simulink model "MPU6050_real_time_Kalman"  (R2023a)
settings: Solver=FixedStepAuto  StartTime=0.0  StopTime=30  RelTol=1e-3
libraries: arduinosensorlib x1
settings Model: ExtModeTrigDuration=2  Creator=admin  LastModifiedBy=admin
settings OptimizationCC: EnhancedBackFolding=on  PassReuseOutputArgsAs=Individual arguments  ZeroExternalMemoryAtStartup=off  ZeroInternalMemoryAtStartup=off  MaxStackSize=64  OptimizeBlockOrder=speed  DifferentSizesBufferReuse=on  OptimizationCustomize=off  EfficientTunableParamExpr=on
settings DebuggingCC: ParameterTunabilityLossMsg=error
settings HardwareCC: ProdBitPerInt=16  ProdBitPerPointer=16  ProdBitPerSizeT=16  ProdBitPerPtrDiffT=16  ProdLargestAtomicFloat=None  ProdWordSize=8  ProdHWDeviceType=Atmel->AVR
settings SFSimCC: MATLABDynamicMemAlloc=off
settings RTWCC: Description=Embedded Coder  SystemTargetFile=ert.tlc  HardwareBoard=Arduino Uno  TemplateMakefile=ert_default_tmf  Toolchain=Arduino AVR
settings CodeAppCC: ForceParamTrailComments=on  IgnoreCustomStorageClasses=off  OperatorAnnotations=on  SimulinkDataObjDesc=on  SFDataObjDesc=on  InsertBlockDesc=on
settings ERTTargetCC: SupportContinuousTime=on  SupportVariableSizeSignals=on  ExtModeTransport=3  ExtModeStaticAlloc=on  ExtModeAutomaticAllocSize=off  ExtModeStaticAllocSize=250  ExtModeMexFile=ext_xcp  ExtModeIntrfLevel=Level2 - Open

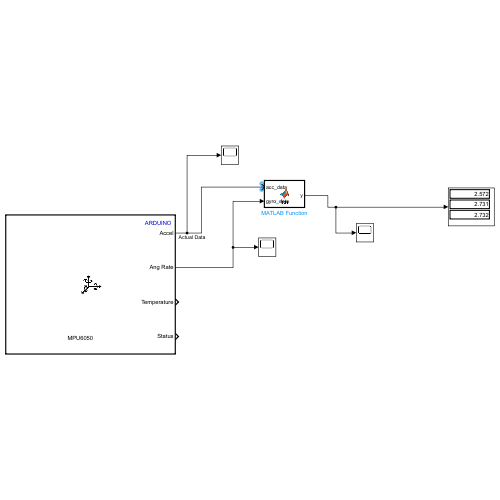
[thumbnail: Simulink's stored preview of the top-level diagram]
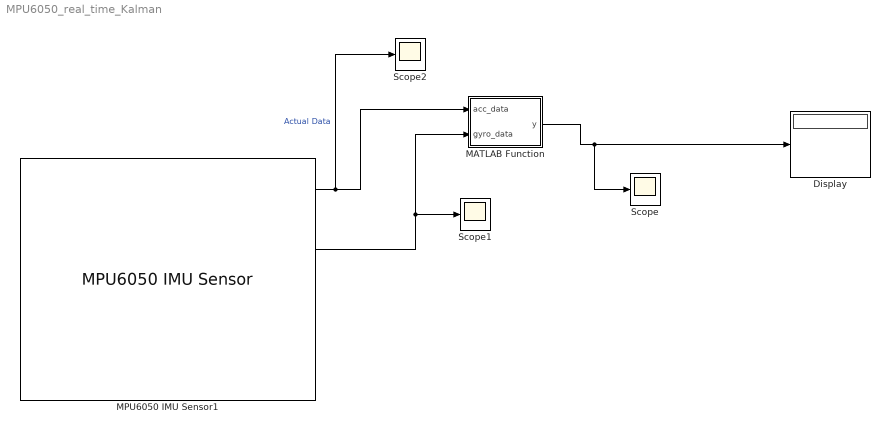
== system MPU6050_real_time_Kalman ==
  Display : Display
  MATLAB Function : MATLAB Function  TreatAsAtomicUnit=on
  MPU6050 IMU Sensor1 : arduinosensorlib/MPU6050 IMU Sensor  SlaveAddress=0x68  Accel=on  AngularRate=on  Temperature=on  Status=on  Timestamp=off  EulerAngles=off  Quat=off  AccelRange=2G  GyroRange=250 dps  DmpOdr=200 Hz  Dlpf=Accelerometer: 184Hz, Gyroscope: 188Hz  spf=1  SampleTime=0.01  QueueSizeFactor=1
  Scope : Scope
  Scope1 : Scope
  Scope2 : Scope
  wires:
  MPU6050 IMU Sensor1/1 -> Scope2/1, MATLAB Function/1(acc_data)  "Actual Data"
  MPU6050 IMU Sensor1/2 -> Scope1/1, MATLAB Function/2(gyro_data)
  MATLAB Function/1(y) -> Scope/1, Display/1

== matlab function MPU6050_real_time_Kalman/MATLAB Function ==
  data: acc_data input; y output; gyro_data input
function y = fcn(acc_data, gyro_data)

    % complementary filter의 가중치 설정
    alpha = 0.95; % 가속도 데이터의 가중치
    dt = 1; % 시간 간격 (임의의 값으로 설정)

    % complementary filter를 적용하여 자세를 결정
    % 가속도 데이터 기반으로 계산
    acc_angle = atan2(acc_data(2), acc_data(1)); % 가속도 데이터를 이용한 각도 추정

    % 자이로 데이터 기반으로 계산
    gyro_angle = gyro_data * dt; % 자이로 데이터를 이용한 각도 변화 추정

    % complementary filter를 사용하여 최종 각도 결정
    y = alpha * acc_angle + (1 - alpha) * gyro_angle;
end
